simulink model "project"  (R2019a)
settings: Solver=FixedStepAuto  StartTime=0.0  StopTime=100  FixedStep=0.001  RelTol=1e-3
libraries: simulink x1
(part 2 of 2)

== matlab function project/Subsystem8/distance direction3 ==
  data: x0 input; y0 input; x1 input; y1 input; x2 input; y2 input; v0x input; v0y input; v1x input; v1y input; a13_x output; a13_y output; v2x input; v2y input
function [ a13_x, a13_y] = fcn(x0, y0, x1, y1, x2, y2, v0x, v0y, v1x,v1y, v2x, v2y)
m=1/10;

k_s= 10;

k_d= 1;

L_r= 1/13;

distance_13_14= sqrt((x1-x2)^2 + (y1-y2)^2);

distance_12_13= sqrt((x1-x0)^2 + (y1-y0)^2);




theta_after= atan2((y1-y2),(x1-x2));
% if x1~=x2
% theta_after= atan2((y1-y2),(x1-x2));
% else
% theta_after= 3.14/2;
% end

f_spring_x_13_14= -k_s* (distance_13_14 - L_r)* cos(theta_after);

f_spring_y_13_14= -k_s* (distance_13_14 - L_r)* sin(theta_after);



theta_before= atan2((y1-y0),(x1-x0));
% if x0~=x1
% theta_before= atan2((y0-y1),(x0-x1));
% else
% theta_before= 3.14/2;
% end

f_spring_x_12_13= -k_s* (distance_12_13 - L_r)* cos(theta_before);

f_spring_y_12_13= -k_s* (distance_12_13 - L_r)* sin(theta_before);






theta_damper_after= atan2((v1y-v2y),(v1x-v2x));
% if v1x~=v2x
% theta_damper_after= atan((v1y-v2y)/(v1x-v2x));
% else
% theta_damper_after= 3.14/2;
% end




damper_force= -k_d * (sqrt((v1y-v2y)^2 + (v1x-v2x)^2));

f_damper_x_13_14 = damper_force *cos(theta_damper_after);
f_damper_y_13_14 = damper_force *sin(theta_damper_after);




theta_damper_before= atan2((v1y-v0y),(v1x-v0x));
% if v0x~=v1x
% theta_damper_before= atan((v0y-v1y)/(v0x-v1x));
% else
% theta_damper_before= 3.14/2;
% end




damper_force_before= -k_d * (sqrt((v0y-v1y)^2 + (v0x-v1x)^2));

f_damper_x_12_13 = damper_force_before *cos(theta_damper_before);
f_damper_y_12_13 = damper_force_before *sin(theta_damper_before);







a13_x = (  f_spring_x_13_14  +   f_damper_x_13_14  + f_spring_x_12_13 + f_damper_x_12_13 )/m;

a13_y = (  f_spring_y_13_14  +   f_damper_y_13_14 + f_spring_y_12_13 + f_damper_y_12_13 + m* (-9.81)  )/m;

== matlab function project/Subsystem9/distance direction3 ==
  data: x0 input; y0 input; x1 input; y1 input; x2 input; y2 input; v0x input; v0y input; v1x input; v1y input; a13_x output; a13_y output; v2x input; v2y input
function [ a13_x, a13_y] = fcn(x0, y0, x1, y1, x2, y2, v0x, v0y, v1x,v1y, v2x, v2y)
m=1/10;

k_s= 10;

k_d= 1;

L_r= 1/13;

distance_13_14= sqrt((x1-x2)^2 + (y1-y2)^2);

distance_12_13= sqrt((x1-x0)^2 + (y1-y0)^2);




theta_after= atan2((y1-y2),(x1-x2));
% if x1~=x2
% theta_after= atan2((y1-y2),(x1-x2));
% else
% theta_after= 3.14/2;
% end

f_spring_x_13_14= -k_s* (distance_13_14 - L_r)* cos(theta_after);

f_spring_y_13_14= -k_s* (distance_13_14 - L_r)* sin(theta_after);



theta_before= atan2((y1-y0),(x1-x0));
% if x0~=x1
% theta_before= atan2((y0-y1),(x0-x1));
% else
% theta_before= 3.14/2;
% end

f_spring_x_12_13= -k_s* (distance_12_13 - L_r)* cos(theta_before);

f_spring_y_12_13= -k_s* (distance_12_13 - L_r)* sin(theta_before);






theta_damper_after= atan2((v1y-v2y),(v1x-v2x));
% if v1x~=v2x
% theta_damper_after= atan((v1y-v2y)/(v1x-v2x));
% else
% theta_damper_after= 3.14/2;
% end




damper_force= -k_d * (sqrt((v1y-v2y)^2 + (v1x-v2x)^2));

f_damper_x_13_14 = damper_force *cos(theta_damper_after);
f_damper_y_13_14 = damper_force *sin(theta_damper_after);




theta_damper_before= atan2((v1y-v0y),(v1x-v0x));
% if v0x~=v1x
% theta_damper_before= atan((v0y-v1y)/(v0x-v1x));
% else
% theta_damper_before= 3.14/2;
% end




damper_force_before= -k_d * (sqrt((v0y-v1y)^2 + (v0x-v1x)^2));

f_damper_x_12_13 = damper_force_before *cos(theta_damper_before);
f_damper_y_12_13 = damper_force_before *sin(theta_damper_before);







a13_x = (  f_spring_x_13_14  +   f_damper_x_13_14  + f_spring_x_12_13 + f_damper_x_12_13 )/m;

a13_y = (  f_spring_y_13_14  +   f_damper_y_13_14 + f_spring_y_12_13 + f_damper_y_12_13 + m* (-9.81)  )/m;
